simulink model "MavlinkTest"  (R2014a)
settings: Solver=FixedStepDiscrete  StartTime=0.0  StopTime=inf  FixedStep=1/30  RelTol=1e-3
InitFcn:
  | load 'busses.mat'
libraries: simulink x4
settings Model: SimulationMode=external  ExtModeTrigDuration=100  Creator=omcaree  LastModifiedBy=omcaree
settings OptimizationCC: OptimizeModelRefInitCode=on  LifeSpan=1
settings DebuggingCC: UnderspecifiedInitializationDetection=Classic  SolverPrmCheckMsg=none
settings HardwareCC: ProdLargestAtomicInteger=Long  ProdLargestAtomicFloat=Double  ProdEndianess=LittleEndian  ProdHWDeviceType=ARM Compatible->ARM Cortex
settings RTWCC: SystemTargetFile=realtime.tlc  GenerateMakefile=off  TemplateMakefile=realtime.tmf  Description=Run on Target Hardware  RTWVerbose=off  ProcessScript=realtime_make_rtw_hook  CustomInclude=include include/common  CustomSource=SerialPort.c
settings RTWCC: CustomHeaderCode=|
  | #include <mavlink.h>
  | #include <common.h>
settings STFCustomTargetCC: TargetLibSuffix=.a  GenerateSampleERTMain=on  ConcurrentExecutionCompliant=off  GeneratePreprocessorConditionals=Use local settings  ERTCustomFileBanners=on  SupportNonInlinedSFcns=off  SupportVariableSizeSignals=on  MATLABClassNameForMDSCustomization=Simulink.SoftwareTarget.ERTCustomization  GRTInterface=off  SystemTargetFile=realtime.tlc
settings ERTTargetCC: CombineOutputUpdateFcns=off  SupportContinuousTime=on  SupportVariableSizeSignals=on  ExtMode=on  ExtModeMexArgs='169.254.0.31' 0 17725 30  ERTSrcFileBannerTemplate=realtime_code_template.cgt  ERTHdrFileBannerTemplate=realtime_code_template.cgt  ERTDataSrcFileTemplate=realtime_code_template.cgt  ERTDataHdrFileTemplate=realtime_code_template.cgt  ERTCustomFileTemplate=realtime_file_process.tlc

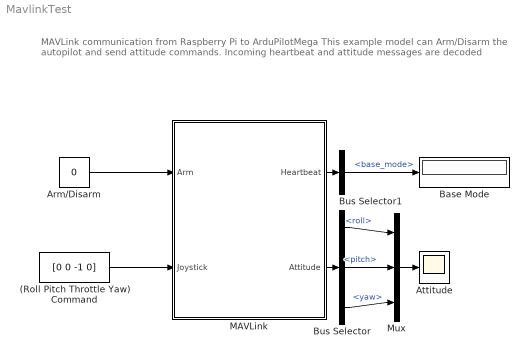
== system MavlinkTest ==
  note: MAVLink communication from Raspberry Pi to ArduPilotMega
      |
      | This example model can Arm/Disarm the autopilot and send attitude commands. Incoming heartbeat and attitude messages are decoded
  (Roll Pitch Throttle Yaw) Command : Constant  Value=[0 0 -1 0]
  Arm/Disarm : Constant  Value=0  OutDataTypeStr=boolean
  Attitude : Scope
      settings: YMin=-0.1  YMax=0.6  SaveName=ScopeData2
  Base Mode : Display
  Bus Selector : BusSelector  OutputSignals=roll,pitch,yaw
  Bus Selector1 : BusSelector  OutputSignals=base_mode
  MAVLink : Subsystem
  Mux : Mux  Inputs=3
  wires:
  MAVLink/2(Attitude) -> Bus Selector/1
  Arm/Disarm/1 -> MAVLink/1(Arm)
  (Roll Pitch Throttle Yaw) Command/1 -> MAVLink/2(Joystick)
  Bus Selector/2 -> Mux/2  "<pitch>"
  Bus Selector/1 -> Mux/1  "<roll>"
  Bus Selector/3 -> Mux/3  "<yaw>"
  Mux/1 -> Attitude/1
  MAVLink/1(Heartbeat) -> Bus Selector1/1
  Bus Selector1/1 -> Base Mode/1  "<base_mode>"

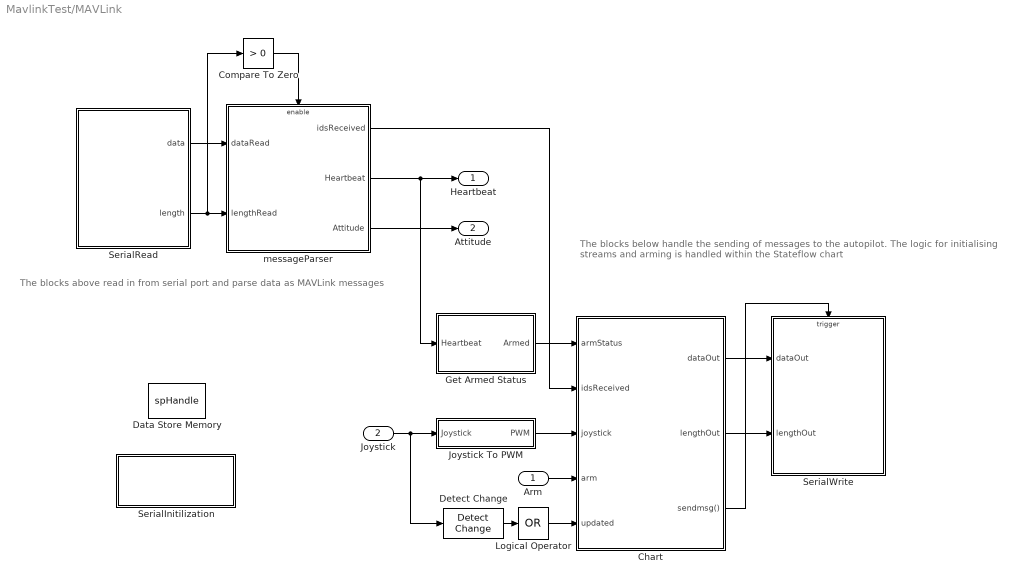
== system MavlinkTest/MAVLink ==
  note: The blocks below handle the sending of messages to the autopilot.
      | The logic for initialising streams and arming is handled within the Stateflow chart
  note: The blocks above read in from serial port and parse data as MAVLink messages
  Arm : Inport  OutDataTypeStr=boolean  PortDimensions=1
  Joystick : Inport  Port=2  PortDimensions=4
  Chart : Stateflow chart  TreatAsAtomicUnit=on
  Compare To Zero : simulink/Logic and Bit Operations/Compare To Zero  relop=>  OutDataTypeStr=boolean
  Data Store Memory : DataStoreMemory  DataStoreName=spHandle  ReadBeforeWriteMsg=warning  WriteAfterWriteMsg=warning  WriteAfterReadMsg=warning  InitialValue=-1  OutDataTypeStr=int32
  Detect Change : simulink/Logic and Bit Operations/Detect Change  vinit=0  InputProcessing=Inherited  OutDataTypeStr=boolean
  Get Armed Status : Subsystem
  Joystick To PWM : Subsystem
  Logical Operator : Logic  Operator=OR  Inputs=1  AllPortsSameDT=off  OutDataTypeStr=boolean
  SerialInitilization : MATLAB Function  TreatAsAtomicUnit=on
  SerialRead : MATLAB Function  TreatAsAtomicUnit=on
  SerialWrite : MATLAB Function  TreatAsAtomicUnit=on
  messageParser : Subsystem
  Heartbeat : Outport
  Attitude : Outport  Port=2
  wires:
  SerialRead/1(data) -> messageParser/1("dataRead ")
  SerialRead/2(length) -> Compare To Zero/1, messageParser/2(lengthRead)
  Chart/1(dataOut) -> SerialWrite/1(dataOut)
  Joystick/1 -> Joystick To PWM/1(Joystick), Detect Change/1
  messageParser/2(Heartbeat) -> Get Armed Status/1(Heartbeat), Heartbeat/1
  Compare To Zero/1 -> messageParser/Enable
  Arm/1 -> Chart/4(arm)
  Chart/2(lengthOut) -> SerialWrite/2(lengthOut)
  messageParser/3(Attitude) -> Attitude/1
  messageParser/1(idsReceived) -> Chart/2(idsReceived)
  Chart/3(sendmsg()) -> SerialWrite/Trigger
  Detect Change/1 -> Logical Operator/1
  Logical Operator/1 -> Chart/5(updated)
  Get Armed Status/1(Armed) -> Chart/1(armStatus)
  Joystick To PWM/1(PWM) -> Chart/3(joystick)

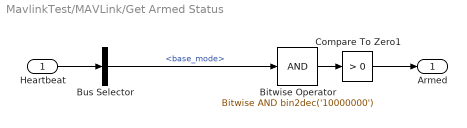
== system MavlinkTest/MAVLink/Get Armed Status ==
  Heartbeat : Inport
  Bitwise Operator : simulink/Logic and Bit Operations/Bitwise Operator  logicop=AND  UseBitMask=on  BitMask=bin2dec('10000000')  BitMaskRealWorld=Stored Integer
  Bus Selector : BusSelector  OutputSignals=base_mode
  Compare To Zero1 : simulink/Logic and Bit Operations/Compare To Zero  relop=>  OutDataTypeStr=boolean
  Armed : Outport
  wires:
  Bitwise Operator/1 -> Compare To Zero1/1
  Compare To Zero1/1 -> Armed/1
  Bus Selector/1 -> Bitwise Operator/1  "<base_mode>"
  Heartbeat/1 -> Bus Selector/1

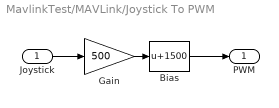
== system MavlinkTest/MAVLink/Joystick To PWM ==
  Joystick : Inport
  Bias : Bias  Bias=1500
  Gain : Gain  Gain=500
  PWM : Outport
  wires:
  Gain/1 -> Bias/1
  Bias/1 -> PWM/1
  Joystick/1 -> Gain/1

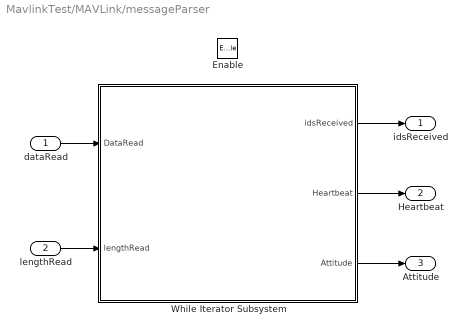
== system MavlinkTest/MAVLink/messageParser ==
  "dataRead " : Inport
  lengthRead : Inport  Port=2
  Enable : EnablePort
  While Iterator Subsystem : Subsystem  TreatAsAtomicUnit=on
  idsReceived : Outport
  Heartbeat : Outport  Port=2
  Attitude : Outport  Port=3
  wires:
  "dataRead "/1 -> While Iterator Subsystem/1(DataRead)
  lengthRead/1 -> While Iterator Subsystem/2(lengthRead)
  While Iterator Subsystem/3(Attitude) -> Attitude/1
  While Iterator Subsystem/2(Heartbeat) -> Heartbeat/1
  While Iterator Subsystem/1("idsReceived ") -> idsReceived/1

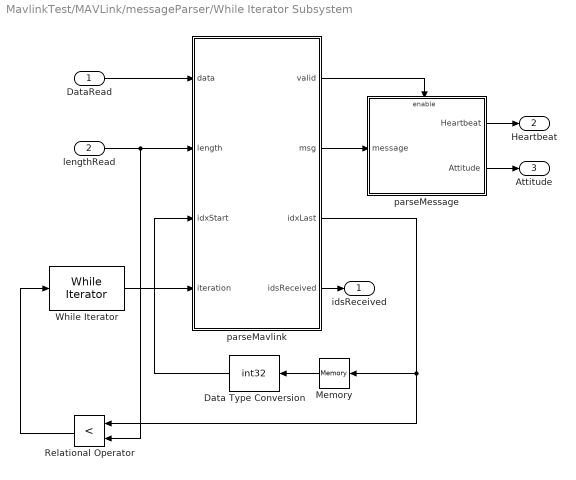
== system MavlinkTest/MAVLink/messageParser/While Iterator Subsystem ==
  DataRead : Inport
  lengthRead : Inport  Port=2
  Data Type Conversion : DataTypeConversion  OutDataTypeStr=int32
  Memory : Memory  X0=1  InheritSampleTime=on
  Relational Operator : RelationalOperator  Operator=<  OutDataTypeStr=boolean
  While Iterator : WhileIterator  MaxIters=100  WhileBlockType=do-while  ShowIterationPort=on
  parseMavlink : MATLAB Function  TreatAsAtomicUnit=on
  parseMessage : Subsystem
  "idsReceived " : Outport
  Heartbeat : Outport  Port=2
  Attitude : Outport  Port=3
  wires:
  DataRead/1 -> parseMavlink/1(data)
  lengthRead/1 -> Relational Operator/2, parseMavlink/2(length)
  Relational Operator/1 -> While Iterator/1
  While Iterator/1 -> parseMavlink/4(iteration)
  Memory/1 -> Data Type Conversion/1
  Data Type Conversion/1 -> parseMavlink/3(idxStart)
  parseMavlink/3(idxLast) -> Relational Operator/1, Memory/1
  parseMavlink/4(idsReceived) -> "idsReceived "/1
  parseMavlink/1(valid) -> parseMessage/Enable
  parseMessage/2(Attitude) -> Attitude/1
  parseMessage/1(Heartbeat) -> Heartbeat/1
  parseMavlink/2(msg) -> parseMessage/1(message)

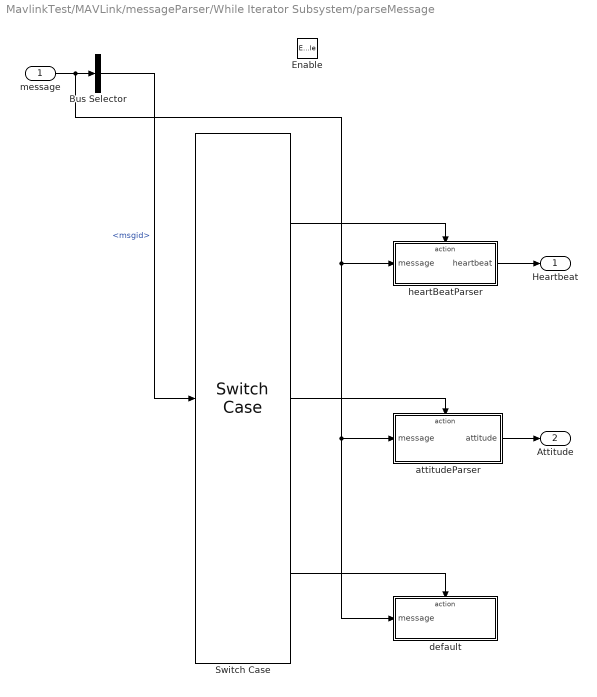
== system MavlinkTest/MAVLink/messageParser/While Iterator Subsystem/parseMessage ==
  message : Inport
  Enable : EnablePort
  Bus Selector : BusSelector  OutputSignals=msgid
  Switch Case : SwitchCase  CaseConditions={0, 30}
  attitudeParser : Subsystem  TreatAsAtomicUnit=on
  default : Subsystem  TreatAsAtomicUnit=on
  heartBeatParser : Subsystem  TreatAsAtomicUnit=on
  Heartbeat : Outport
  Attitude : Outport  Port=2
  wires:
  message/1 -> heartBeatParser/1(message), default/1(message), attitudeParser/1(message), Bus Selector/1
  Switch Case/2 -> attitudeParser/Action
  Switch Case/1 -> heartBeatParser/Action
  heartBeatParser/1(heartbeat) -> Heartbeat/1
  attitudeParser/1(attitude) -> Attitude/1
  Bus Selector/1 -> Switch Case/1  "<msgid>"
  Switch Case/3 -> default/Action

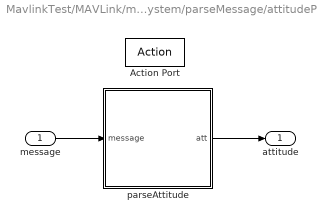
== system MavlinkTest/MAVLink/messageParser/While Iterator Subsystem/parseMessage/attitudeParser ==
  message : Inport
  Action Port : ActionPort  ActionType=case
  parseAttitude : MATLAB Function  TreatAsAtomicUnit=on
  attitude : Outport
  wires:
  message/1 -> parseAttitude/1(message)
  parseAttitude/1(att) -> attitude/1

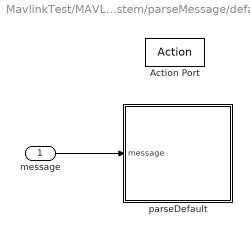
== system MavlinkTest/MAVLink/messageParser/While Iterator Subsystem/parseMessage/default ==
  message : Inport
  Action Port : ActionPort  ActionType=default
  parseDefault : MATLAB Function  TreatAsAtomicUnit=on
  wires:
  message/1 -> parseDefault/1(message)

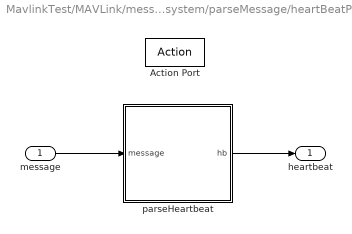
== system MavlinkTest/MAVLink/messageParser/While Iterator Subsystem/parseMessage/heartBeatParser ==
  message : Inport
  Action Port : ActionPort  ActionType=case
  parseHeartbeat : MATLAB Function  TreatAsAtomicUnit=on
  heartbeat : Outport
  wires:
  parseHeartbeat/1(hb) -> heartbeat/1
  message/1 -> parseHeartbeat/1(message)

== matlab function MavlinkTest/MAVLink/messageParser/While Iterator Subsystem/parseMavlink ==
  data: valid output; data input; msg output Bus: message; length input; idxStart input; idxLast output; iteration input; idsReceived output size=256
function [valid,msg,idxLast,idsReceived]  = parseMavlink(data, length, idxStart,iteration)

status = struct(...
    'msg_received', uint8(0),...
    'buffer_overrun', uint8(0),...
    'parse_error', uint8(0),...
    'parse_state', int32(0),...
    'packet_idx', uint8(0),...
    'current_rx_seq', uint8(0),...
    'current_tx_seq', uint8(0),...
    'packet_rx_success_count', uint16(0),...
    'packet_rx_drop_count', uint16(0));
persistent message;
if isempty(message)
    message = struct(...
        'checksum', uint16(0),...
        'magic', uint8(0),...
        'len', uint8(0),...
        'seq', uint8(0),...
        'sysid', uint8(0),...
        'compid', uint8(0),...
        'msgid', uint8(0),...
        'payload64', zeros(33*2,1,'uint32'));
end

valid = uint8(0);
idxLast=int32(1);

persistent ids;
if isempty(ids)
   ids=zeros(256,1,'uint8'); 
end
if iteration==1
    idxStart=iteration;
    ids=zeros(256,1,'uint8');
end
if ~coder.target('SFun')
    for i=idxStart:length
        valid=uint8(0);
        valid=coder.ceval('mavlink_parse_char',0,data(i),coder.ref(message),coder.ref(status));         
        if valid>0
            ids(message.msgid+1)=uint8(1);
            if i==length
                idxLast=i;
            else
                idxLast=i+1;
            end            
            break;
        else
            idxLast=i;% if itteration finishes without id trigger - 
        end         
    end     
end
idsReceived=ids;
msg = message;

== matlab function MavlinkTest/MAVLink/SerialWrite ==
  data: dataOut input uint8; lengthOut input; spHandle data_store_memory
  events: trigger input FUNCTION_CALL_EVENT
function serialWrite(dataOut, lengthOut)
global spHandle;
if ~coder.target('SFun')  
        if lengthOut>0           
            coder.ceval('write',spHandle, coder.ref(dataOut), uint32(lengthOut));
        end   
end

== matlab function MavlinkTest/MAVLink/messageParser/While Iterator Subsystem/parseMessage/default/parseDefault ==
  data: message input
function parseDefault(message)

if ~coder.target('SFun')
    fprintf('Unhandled message received (ID: %d)\n',int16(message.msgid));
end

== matlab function MavlinkTest/MAVLink/messageParser/While Iterator Subsystem/parseMessage/attitudeParser/parseAttitude ==
  data: att output Bus: attitude; message input
function att = parseAttitude(message)

att.time_boot_ms = uint32(0);
att.roll = single(0);
att.pitch = single(0);
att.yaw = single(0);
att.rollspeed = single(0);
att.pitchspeed = single(0);
att.yawspeed = single(0);

if ~coder.target('SFun')
    coder.ceval('mavlink_msg_attitude_decode',coder.ref(message),coder.ref(att));
end

== stateflow chart MavlinkTest/MAVLink/Chart ==
  note: Note: idsReceived are incremented by 1 as Simulink is one-based
      | Therefore heartbeat (0) is 1 and attitude (30) is 31
  state Initializing
    state EstablishingConnection
      en:hbCount=1;
      du:if idsReceived(1)==1 hbCount=hbCount+1; end
    note: Wait for 5 heatbeats to
        | make sure autopilot is alive
    state requestingAttitude
      entry:
      [dataOut,lengthOut] = requestStream(uint8(10),uint8(50));
      send(sendmsg);
    note: Request the attitude message every
        | second, until it is received
    (default) -> EstablishingConnection
    EstablishingConnection -> requestingAttitude : [hbCount==5]
    requestingAttitude -> requestingAttitude [order 2] : after(1,sec)
  state Disarm
    entry:
    [dataOut,lengthOut] = sendArmDisarm(0);
    send(sendmsg);
  state Arm
    entry:
    [dataOut,lengthOut] = sendArmDisarm(1);
    send(sendmsg);
  state Sky
    during:
    if updated
    [dataOut,lengthOut] =sendRCOverride(joystick);
    send(sendmsg);
    end
  (default) -> Initializing
  requestingAttitude -> Disarm [order 1] : [idsReceived(31)==1]
  Disarm -> Disarm [order 2] : after(1,sec)[armStatus]
  Sky -> Disarm : [~arm || ~armStatus]
  Disarm -> Arm [order 1] : [arm]
  Arm -> Arm [order 2] : after(5,sec)[~armStatus]
  Arm -> Sky [order 1] : [armStatus]
  data: data function_output; length function_output; streamId function_input; rate function_input; data function_output; length function_output; armdisarm function_input; data function_output; length function_output; js function_input; dataOut output; lengthOut output; armStatus input size=1; idsReceived input size=256; hbCount local; joystick input; arm input boolean; updated input
  events: sendmsg output FUNCTION_CALL_EVENT
  function [data,length] = requestStream(streamId, rate):
    | function [data,length] = requestStream(streamId, rate)
    | data2 = zeros(256,1,'uint8');
    | length = uint8(0);
    | 
    | message = struct(...
    |     'checksum', uint16(0),...
    |     'magic', uint8(0),...
    |     'len', uint8(0),...
    |     'seq', uint8(0),...
    |     'sysid', uint8(0),...
    |     'compid', uint8(0),...
    |     'msgid', uint8(0),...
    |     'payload64', zeros(33*2,1,'uint32'));
    | 
    | if ~coder.target('SFun')
    |   coder.ceval('mavlink_msg_request_data_stream_pack',...
    |       255,0,coder.ref(message),1,0,uint8(streamId),uint8(rate),1);
    |   length = message.len+8;
    |   coder.ceval('mavlink_msg_to_send_buffer',...
    |       coder.ref(data2),coder.ref(message));
    | end
    | data=data2;
  function [data,length] = sendArmDisarm(armdisarm):
    | function  [data,length] = sendArmDisarm(armdisarm)
    | data2 = zeros(256,1,'uint8');
    | length = uint8(0);
    | 
    | message = struct(...
    |     'checksum', uint16(0),...
    |     'magic', uint8(0),...
    |     'len', uint8(0),...
    |     'seq', uint8(0),...
    |     'sysid', uint8(0),...
    |     'compid', uint8(0),...
    |     'msgid', uint8(0),...
    |     'payload64', zeros(33*2,1,'uint32'));
    | 
    | if ~coder.target('SFun')
    |   coder.ceval('mavlink_msg_command_long_pack',...
    |       255,0,coder.ref(message),1,250,400,0,uint8(armdisarm),0,0,0,0,0,0);
    |   length = message.len+8;
    |   coder.ceval('mavlink_msg_to_send_buffer',...
    |       coder.ref(data2),coder.ref(message));
    | end
    | data=data2;
  function [data,length] = sendRCOverride(js):
    | function [data,length] = sendRCOverride(js)
    | data2 = zeros(256,1,'uint8');
    | length = uint8(0);
    | 
    | message = struct(...
    |     'checksum', uint16(0),...
    |     'magic', uint8(0),...
    |     'len', uint8(0),...
    |     'seq', uint8(0),...
    |     'sysid', uint8(0),...
    |     'compid', uint8(0),...
    |     'msgid', uint8(0),...
    |     'payload64', zeros(33*2,1,'uint32'));
    | 
    | if ~coder.target('SFun')
    |   coder.ceval('mavlink_msg_rc_channels_override_pack',...
    |       255,0,coder.ref(message),1,0,uint16(js(1)),uint16(js(2)),...
    |       uint16(js(3)),uint16(js(4)),0,0,0,0);
    |   length = message.len+8;
    |   coder.ceval('mavlink_msg_to_send_buffer',...
    |       coder.ref(data2),coder.ref(message));
    | end
    | data=data2;

== matlab function MavlinkTest/MAVLink/SerialRead ==
  data: data output; length output; spHandle data_store_memory
function [data,length]=serialRead
global spHandle;
data = zeros(512,1,'uint8');
length =int32(0);
if ~coder.target('SFun')
    if spHandle>0
        bytesRead = int32(0);
        dataRead = zeros(512,1,'uint8');
        bytesRead = coder.ceval('read',spHandle, coder.ref(dataRead), uint32(512));
        if bytesRead>0
            data= dataRead;
            length=bytesRead;
        end
    end
end

== matlab function MavlinkTest/MAVLink/SerialInitilization ==
  data: spHandle data_store_memory
function initSerial
global spHandle;
if ~coder.target('SFun')   
    if isempty(spHandle)||spHandle==-1;
        spHandle=int32(0);
        spHandle =coder.ceval('setupSerialPort',['/dev/ttyAMA0' 0], uint32(57600));
    end 
end

== matlab function MavlinkTest/MAVLink/messageParser/While Iterator Subsystem/parseMessage/heartBeatParser/parseHeartbeat ==
  data: hb output Bus: heartbeat; message input
function hb = parseHeartbeat(message)

 hb.custom_mode = uint32(0);
 hb.type = uint8(0);
 hb.autopilot = uint8(0);
 hb.base_mode = uint8(0);
 hb.system_status = uint8(0);
 hb.mavlink_version = uint8(0);

if ~coder.target('SFun')
    coder.ceval('mavlink_msg_heartbeat_decode', coder.ref(message), coder.ref(hb)); 
end
